simulink model "B1P15_Torsonal_Model_From_V_Rizzo_One_Coupler"  (Simulink 7.5)
settings: Solver=ode23tb  StartTime=0.0  StopTime=0.5  RelTol=1e-3
InitFcn:
  | B1P15_Torsonal_Model_From_V_Rizzo_One_Coupler_Constants
values from neighbouring files (symbols this model uses):
  Ka = 10    [B1P15_Torsonal_Model_From_V_Rizzo_One_Coupler_Constants.m]    (also in RizzoConst.m)
  Ke = 10    [B1P15_Torsonal_Model_From_V_Rizzo_One_Coupler_Constants.m]    (also in RizzoConst.m)
  Kr = 10    [B1P15_Torsonal_Model_From_V_Rizzo_One_Coupler_Constants.m]    (also in RizzoConst.m)
  Kt = 10    [B1P15_Torsonal_Model_From_V_Rizzo_One_Coupler_Constants.m]    (also in RizzoConst.m)
  Ms = 1/((Jm+JL)*s*F)    [B1P15_Torsonal_Model_From_V_Rizzo_One_Coupler_Constants.m]
  R = 10    [B1P15_Torsonal_Model_From_V_Rizzo_One_Coupler_Constants.m]    (also in RizzoConst.m)
settings Model: Creator=geovana  LastModifiedBy=geovana
settings OptimizationCC: InitFltsAndDblsToZero=on
settings DebuggingCC: SaveWithParameterizedLinksMsg=none  SignalResolutionControl=TryResolveAllWithWarning  MultiTaskDSMMsg=warning  MultiTaskCondExecSysMsg=none  StrictBusMsg=Warning
settings RTWCC: IncludeERTFirstTime=on
settings GRTTargetCC: TargetFcnLib=ansi_tfl_tmw.mat

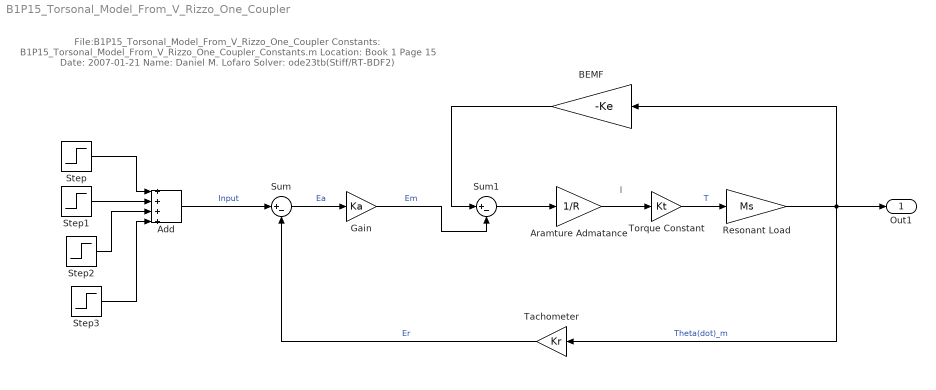
== system B1P15_Torsonal_Model_From_V_Rizzo_One_Coupler ==
  note: File:B1P15_Torsonal_Model_From_V_Rizzo_One_Coupler
      | Constants: B1P15_Torsonal_Model_From_V_Rizzo_One_Coupler_Constants.m
      | Location: Book 1 Page 15
      | Date: 2007-01-21
      | Name: Daniel M. Lofaro
      | Solver: ode23tb(Stiff/RT-BDF2)
  note: I
  Add : Sum  Inputs=++++  OutDataType=sfix(16)  OutScaling=2^-10
  Aramture Admatance : Gain  Gain=1/R  ParameterDataType=sfix(16)  ParameterScaling=2^0  OutDataType=sfix(16)  OutScaling=2^0
  BEMF : Gain  Gain=-Ke  ParameterDataType=sfix(16)  ParameterScaling=2^0  OutDataType=sfix(16)  OutScaling=2^0
  Gain : Gain  Gain=Ka  ParameterDataType=sfix(16)  ParameterScaling=2^0  OutDataType=sfix(16)  OutScaling=2^0
  Resonant Load : Gain  Gain=Ms  ParameterDataType=sfix(16)  ParameterScaling=2^0  OutDataType=sfix(16)  OutScaling=2^0
  Step : Step  Time=0.1  SampleTime=0
  Step1 : Step  Time=0.2  After=-1  SampleTime=0
  Step2 : Step  Time=0.3  After=-1  SampleTime=0
  Step3 : Step  Time=0.4  SampleTime=0
  Sum : Sum  Inputs=|+-  OutDataType=sfix(16)  OutScaling=2^0
  Sum1 : Sum  Inputs=|+-  OutDataType=sfix(16)  OutScaling=2^0
  Tachometer : Gain  Gain=Kr  ParameterDataType=sfix(16)  ParameterScaling=2^0  OutDataType=sfix(16)  OutScaling=2^0
  Torque Constant : Gain  Gain=Kt  ParameterDataType=sfix(16)  ParameterScaling=2^0  OutDataType=sfix(16)  OutScaling=2^0
  Out1 : Outport  OutDataType=sfix(16)  OutScaling=2^0
  wires:
  Step/1 -> Add/1
  Step1/1 -> Add/2
  Step2/1 -> Add/3
  Step3/1 -> Add/4
  Add/1 -> Sum/1  "Input"
  Sum/1 -> Gain/1  "Ea"
  Sum1/1 -> Aramture Admatance/1
  Aramture Admatance/1 -> Torque Constant/1
  Torque Constant/1 -> Resonant Load/1  "T"
  BEMF/1 -> Sum1/1
  Gain/1 -> Sum1/2  "Em"
  Tachometer/1 -> Sum/2  "Er"
  Resonant Load/1 -> Out1/1, BEMF/1, Tachometer/1  "Theta(dot)_m"
